simulink library "hcu_lib"  (Simulink 8.6)
settings: Solver=ode45  SolverMode=SingleTasking  StartTime=0.0  StopTime=10.0  RelTol=1e-3
PreLoadFcn:
  | if exist('tl_preloadfcn','file'), tl_preloadfcn(gcs,100); end
PostLoadFcn:
  | if exist('tl_postloadfcn','file'), tl_postloadfcn(gcs,100); end
undefined symbols (not defined in the file or in its folder): C_TICK_TIME_S, DEG2RAD, EPSILON, FALSE, RAD2DEG, TRUE
undefined symbols (not defined in the file): UNDEFINED_VALUE
libraries: hcu_lib x19, simulink x4
(part 3 of 3)

== stateflow chart Derivative/Function Call Generator ==
  (default) -> (junction 63)
  (junction 63) -> (junction 64) [order 1] : [SampleTime_S<=C_TICK_TIME_S]
  (junction 63) -> (junction 65) [order 2] : {Timer=Timer+C_TICK_TIME_S;}
  (junction 64) -> (junction 67) : {FunCall;}
  (junction 65) -> (junction 66) [order 1] : [Timer>=SampleTime_S-0.0001]
  (junction 65) -> (junction 69) [order 2]
  (junction 66) -> (junction 68) : {FunCall;}
  (junction 67) -> (junction 71) : {Timer=0;}
  (junction 68) -> (junction 70) : {Timer=0;}
  (junction 70) -> (junction 69)
  (junction 71) -> (junction 70)
  data: SampleTime_S input double; C_TICK_TIME_S parameter double; Timer local single
  events: FunCall output FUNCTION_CALL_EVENT

== stateflow chart latching_fault_filter/lff_ctl ==
  (default) -> (junction 92)
  (junction 92) -> (junction 93) [order 1] : [i_fault]
      | {count+=inc;}
  (junction 92) -> (junction 93) [order 2] : {count-=dec;}
  (junction 93) -> (junction 94)
  (junction 94) -> (junction 95) [order 1] : [count>=sat]
      | {count=sat;
      | fault_flg=1;}
  (junction 94) -> (junction 95) [order 2] : [count<=0]
      | {count=0;}
  (junction 94) -> (junction 95) [order 3]
  (junction 95) -> (junction 96) : {ff_count = count;}
  data: sat input uint8; inc input uint8; dec input uint8; i_fault input boolean; fault_flg output boolean =0; ff_count output uint8; count local int16 =0
